simulink model "Consensus_HP"  (R2022b)
settings: Solver=VariableStepAuto  StartTime=0.0  StopTime=20  RelTol=1e-3
undefined symbols (not defined in the file): N
libraries: cstblocks x4
settings Model: Creator=Lirui  LastModifiedBy=ROG
settings ModelReferenceCC: EnableRefExpFcnMdlSchedulingChecks=on

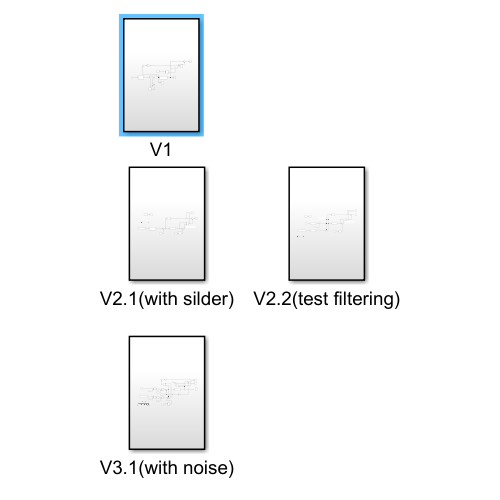
[thumbnail: Simulink's stored preview of the top-level diagram]
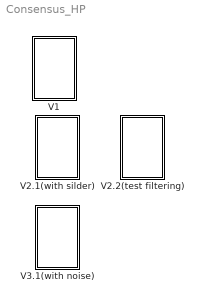
== system Consensus_HP ==
  V1 : Subsystem
  V2.1(with silder) : Subsystem
  V2.2(test filtering) : Subsystem
  V3.1(with noise) : Subsystem

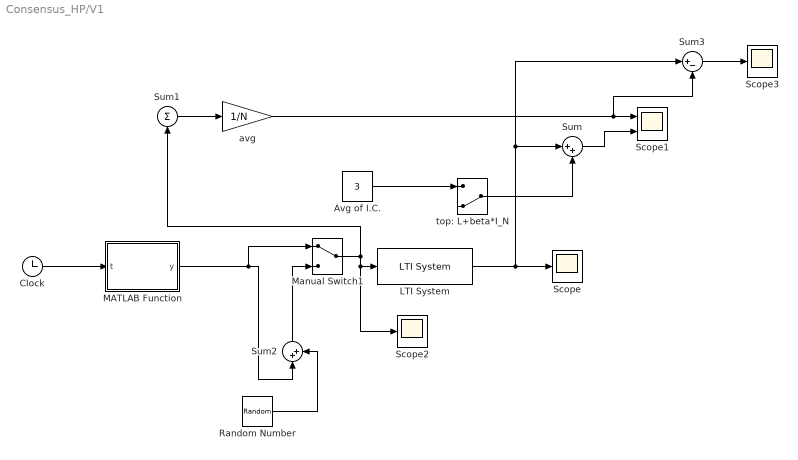
== system Consensus_HP/V1 ==
  Avg of I.C. : Constant  Value=3
  Clock : Clock
  LTI System : cstblocks/LTI System  sys=H  IC=[]
  MATLAB Function : MATLAB Function  TreatAsAtomicUnit=on
  Manual Switch1 : ManualSwitch
  Random Number : RandomNumber  Mean=0*ones(N,1)  Variance=[0.01 0.02 0.03 0.04]'
  Scope : Scope
  Scope1 : Scope  NumInputPorts=2
  Scope2 : Scope
  Scope3 : Scope
  Sum : Sum  Inputs=|++
  Sum1 : Sum  Inputs=|+
  Sum2 : Sum  Inputs=|++
  Sum3 : Sum  Inputs=|+-
  avg : Gain  Gain=1/N
  top: L+beta*I_N : ManualSwitch  CurrentSetting=0
  wires:
  avg/1 -> Scope1/1, Sum3/2
  LTI System/1 -> Sum3/1, Sum/1, Scope/1
  Sum1/1 -> avg/1
  Sum/1 -> Scope1/2
  Clock/1 -> MATLAB Function/1(t)
  MATLAB Function/1(y) -> Manual Switch1/1, Sum2/1
  top: L+beta*I_N/1 -> Sum/2
  Avg of I.C./1 -> top: L+beta*I_N/1
  Random Number/1 -> Sum2/2
  Manual Switch1/1 -> Sum1/1, Scope2/1, LTI System/1
  Sum2/1 -> Manual Switch1/2
  Sum3/1 -> Scope3/1

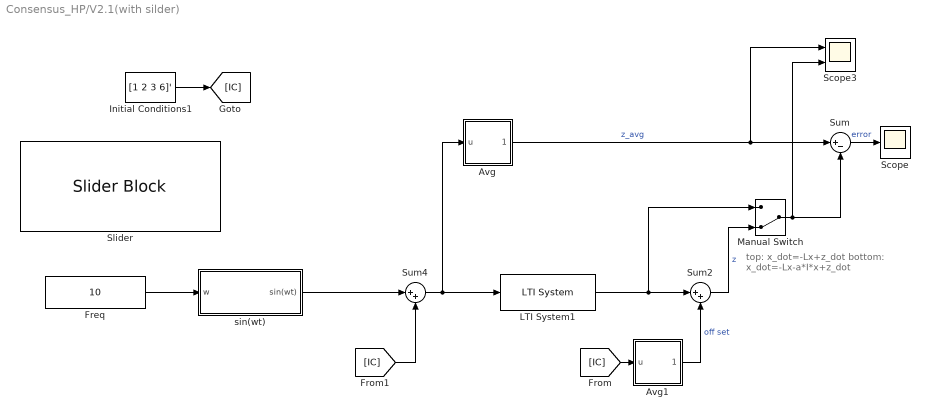
== system Consensus_HP/V2.1(with silder) ==
  note: top:       x_dot=-Lx+z_dot
      | bottom: x_dot=-Lx-a*I*x+z_dot
  Avg : Subsystem
  Avg1 : Subsystem
  Freq : Constant  Value=10
  Initial Conditions1 : Constant  Value=[1 2 3 6]'
  LTI System1 : cstblocks/LTI System  sys=H  IC=[]
  Manual Switch : ManualSwitch  CurrentSetting=0
  Scope : Scope
  Scope3 : Scope  NumInputPorts=2
  Slider : SliderBlock  ScaleMin=0.001  ScaleMax=10  ScaleType=Log
  Sum : Sum  Inputs=|+-
  Sum2 : Sum  Inputs=|++
  Sum4 : Sum  Inputs=|++
  sin(wt) : Subsystem
  wires:
  LTI System1/1 -> Manual Switch/1, Sum2/1
  [IC] -> Sum4/2
  Sum4/1 -> Avg/1(u), LTI System1/1
  Sum/1 -> Scope/1  "error"
  Avg/1(avg(u)) -> Sum/1, Scope3/1  "z_avg"
  Freq/1 -> sin(wt)/1(w)
  sin(wt)/1(sin(wt)) -> Sum4/1
  Avg1/1(avg(u)) -> Sum2/2  "off set"
  Manual Switch/1 -> Scope3/2, Sum/2
  Sum2/1 -> Manual Switch/2  "z"
  Initial Conditions1/1 -> [IC]
  [IC] -> Avg1/1(u)

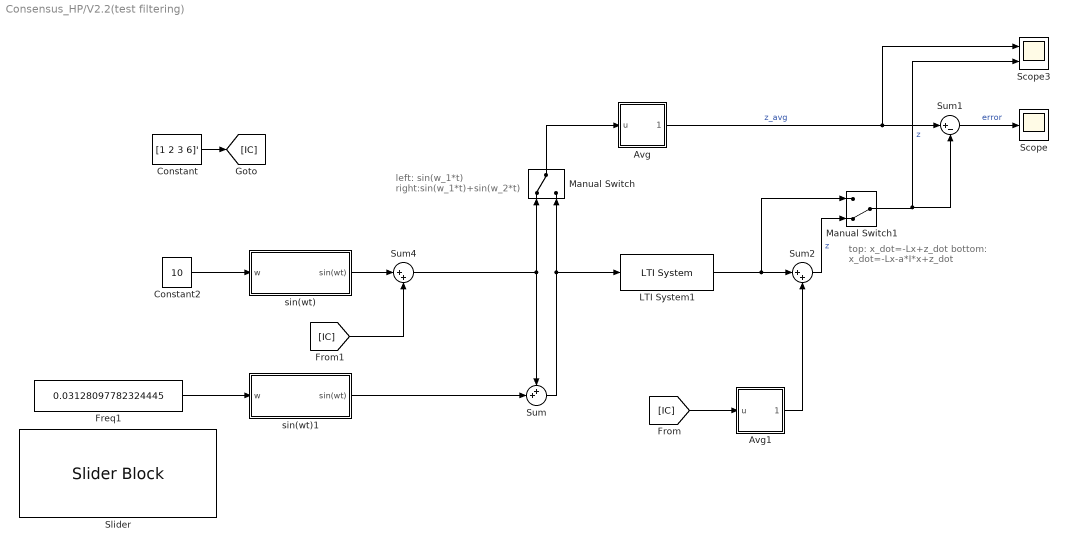
== system Consensus_HP/V2.2(test filtering) ==
  note: left:  sin(w_1*t)
      | right:sin(w_1*t)+sin(w_2*t)
  note: top:       x_dot=-Lx+z_dot
      | bottom: x_dot=-Lx-a*I*x+z_dot
  Avg : Subsystem
  Avg1 : Subsystem
  Constant : Constant  Value=[1 2 3 6]'
  Constant2 : Constant  Value=10
  Freq1 : Constant  Value=0.03128097782324445
  LTI System1 : cstblocks/LTI System  sys=H  IC=[]
  Manual Switch : ManualSwitch
  Manual Switch1 : ManualSwitch  CurrentSetting=0
  Scope : Scope
  Scope3 : Scope  NumInputPorts=2
  Slider : SliderBlock  ScaleMin=0.001  ScaleType=Log
  Sum : Sum  Inputs=++|
  Sum1 : Sum  Inputs=|+-
  Sum2 : Sum  Inputs=|++
  Sum4 : Sum  Inputs=|++
  sin(wt) : Subsystem
  sin(wt)1 : Subsystem
  wires:
  LTI System1/1 -> Manual Switch1/1, Sum2/1
  [IC] -> Sum4/2
  sin(wt)/1(sin(wt)) -> Sum4/1
  Sum4/1 -> Manual Switch/1, Sum/1
  Sum/1 -> LTI System1/1, Manual Switch/2
  Constant2/1 -> sin(wt)/1(w)
  sin(wt)1/1(sin(wt)) -> Sum/2
  Freq1/1 -> sin(wt)1/1(w)
  Avg/1(avg(u)) -> Sum1/1, Scope3/1  "z_avg"
  Manual Switch/1 -> Avg/1(u)
  Constant/1 -> [IC]
  [IC] -> Avg1/1(u)
  Avg1/1(avg(u)) -> Sum2/2
  Sum2/1 -> Manual Switch1/2  "z"
  Manual Switch1/1 -> Sum1/2, Scope3/2  "z"
  Sum1/1 -> Scope/1  "error"

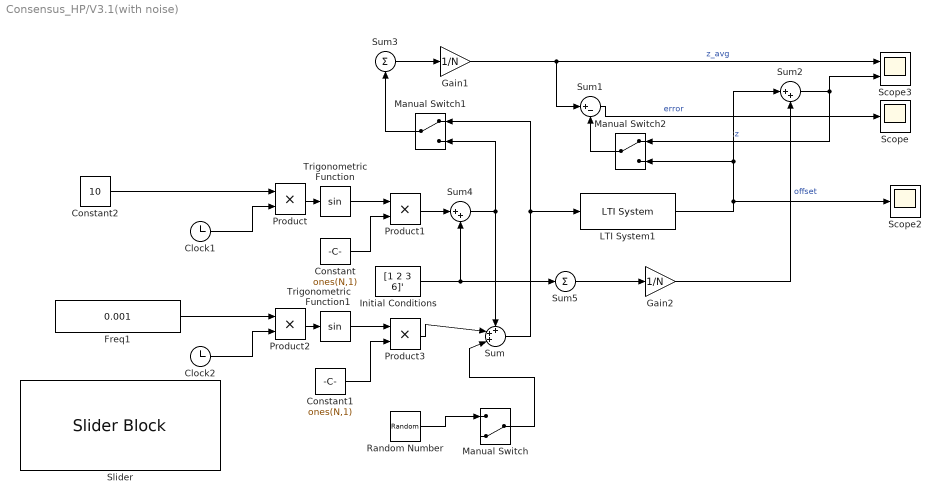
== system Consensus_HP/V3.1(with noise) ==
  Clock1 : Clock
  Clock2 : Clock
  Constant : Constant  Value=ones(N,1)
  Constant1 : Constant  Value=ones(N,1)
  Constant2 : Constant  Value=10
  Freq1 : Constant  Value=0.001
  Gain1 : Gain  Gain=1/N
  Gain2 : Gain  Gain=1/N
  Initial Conditions : Constant  Value=[1 2 3 6]'
  LTI System1 : cstblocks/LTI System  sys=H  IC=[]
  Manual Switch : ManualSwitch  CurrentSetting=0
  Manual Switch1 : ManualSwitch
  Manual Switch2 : ManualSwitch
  Product{,1..3} (4 alike) : Product
  Random Number : RandomNumber  Mean=0*ones(N,1)  Variance=[0.1 0.1 0.1 0.1]'
  Scope : Scope
  Scope2 : Scope
  Scope3 : Scope  NumInputPorts=2
  Slider : SliderBlock  ScaleMin=0.001  ScaleType=Log
  Sum : Sum  Inputs=+++|
  Sum1 : Sum  Inputs=|+-
  Sum2 : Sum  Inputs=|++
  Sum3 : Sum  Inputs=|+
  Sum4 : Sum  Inputs=|++
  Sum5 : Sum  Inputs=+
  Trigonometric Function : Trigonometry
  Trigonometric Function1 : Trigonometry
  wires:
  Gain2/1 -> Sum2/2  "offset"
  Trigonometric Function/1 -> Product1/1
  LTI System1/1 -> Scope2/1, Manual Switch2/2, Sum2/1
  Constant/1 -> Product1/2
  Constant2/1 -> Product/1
  Gain1/1 -> Scope3/1, Sum1/1  "z_avg"
  Sum2/1 -> Manual Switch2/1, Scope3/2  "z"
  Product/1 -> Trigonometric Function/1
  Initial Conditions/1 -> Sum5/1, Sum4/2
  Clock1/1 -> Product/2
  Product1/1 -> Sum4/1
  Sum4/1 -> Manual Switch1/2, Sum/1
  Sum5/1 -> Gain2/1
  Sum3/1 -> Gain1/1
  Product2/1 -> Trigonometric Function1/1
  Clock2/1 -> Product2/2
  Constant1/1 -> Product3/2
  Trigonometric Function1/1 -> Product3/1
  Freq1/1 -> Product2/1
  Product3/1 -> Sum/2
  Sum/1 -> Manual Switch1/1, LTI System1/1
  Random Number/1 -> Manual Switch/1
  Manual Switch/1 -> Sum/3
  Manual Switch1/1 -> Sum3/1
  Sum1/1 -> Scope/1  "error"
  Manual Switch2/1 -> Sum1/2

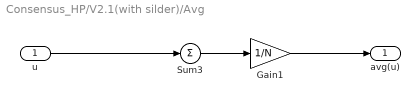
== system Consensus_HP/V2.1(with silder)/Avg ==
  u : Inport
  Gain1 : Gain  Gain=1/N
  Sum3 : Sum  Inputs=+
  avg(u) : Outport
  wires:
  Sum3/1 -> Gain1/1
  u/1 -> Sum3/1
  Gain1/1 -> avg(u)/1

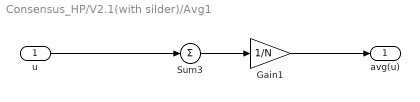
== system Consensus_HP/V2.1(with silder)/Avg1 ==
  u : Inport
  Gain1 : Gain  Gain=1/N
  Sum3 : Sum  Inputs=+
  avg(u) : Outport
  wires:
  Sum3/1 -> Gain1/1
  u/1 -> Sum3/1
  Gain1/1 -> avg(u)/1

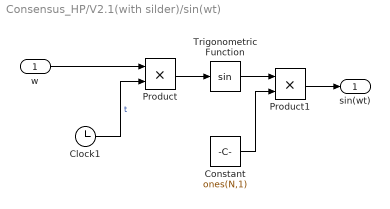
== system Consensus_HP/V2.1(with silder)/sin(wt) ==
  w : Inport
  Clock1 : Clock
  Constant : Constant  Value=ones(N,1)
  Product : Product
  Product1 : Product
  Trigonometric Function : Trigonometry
  sin(wt) : Outport
  wires:
  w/1 -> Product/1
  Product/1 -> Trigonometric Function/1
  Clock1/1 -> Product/2  "t"
  Product1/1 -> sin(wt)/1
  Trigonometric Function/1 -> Product1/1
  Constant/1 -> Product1/2

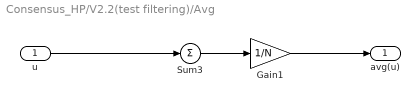
== system Consensus_HP/V2.2(test filtering)/Avg ==
  u : Inport
  Gain1 : Gain  Gain=1/N
  Sum3 : Sum  Inputs=+
  avg(u) : Outport
  wires:
  Sum3/1 -> Gain1/1
  u/1 -> Sum3/1
  Gain1/1 -> avg(u)/1

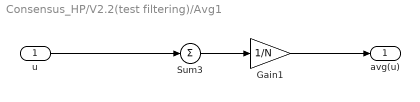
== system Consensus_HP/V2.2(test filtering)/Avg1 ==
  u : Inport
  Gain1 : Gain  Gain=1/N
  Sum3 : Sum  Inputs=+
  avg(u) : Outport
  wires:
  Sum3/1 -> Gain1/1
  u/1 -> Sum3/1
  Gain1/1 -> avg(u)/1

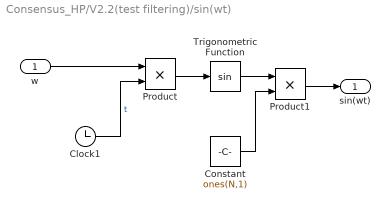
== system Consensus_HP/V2.2(test filtering)/sin(wt) ==
  w : Inport
  Clock1 : Clock
  Constant : Constant  Value=ones(N,1)
  Product : Product
  Product1 : Product
  Trigonometric Function : Trigonometry
  sin(wt) : Outport
  wires:
  w/1 -> Product/1
  Product/1 -> Trigonometric Function/1
  Clock1/1 -> Product/2  "t"
  Product1/1 -> sin(wt)/1
  Trigonometric Function/1 -> Product1/1
  Constant/1 -> Product1/2

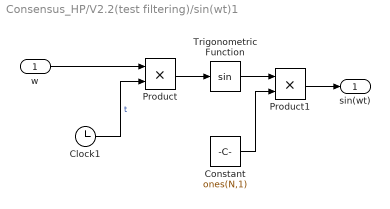
== system Consensus_HP/V2.2(test filtering)/sin(wt)1 ==
  w : Inport
  Clock1 : Clock
  Constant : Constant  Value=ones(N,1)
  Product : Product
  Product1 : Product
  Trigonometric Function : Trigonometry
  sin(wt) : Outport
  wires:
  w/1 -> Product/1
  Product/1 -> Trigonometric Function/1
  Clock1/1 -> Product/2  "t"
  Product1/1 -> sin(wt)/1
  Trigonometric Function/1 -> Product1/1
  Constant/1 -> Product1/2

== matlab function Consensus_HP/V1/MATLAB Function ==
  data: t input; y output
function y = fcn(t)
w=10;
%y=[sin(w*t)+1,sin(w*t)+2,sin(w*t)+3,sin(w*t)+6]';

%y=[exp(-t)+1,exp(-t)+2,exp(-t)+3,exp(-t)+6]';


%y=[ 1,2,3,6]';
y=[0,2,2,2]';
